simulink model "Practica2"  (R2019a)
settings: Solver=VariableStepAuto  StartTime=0.0  StopTime=10.0  RelTol=1e-3
undefined symbols (not defined in the file or in its folder): k
settings Model: Creator=Andres  LastModifiedBy=Andres

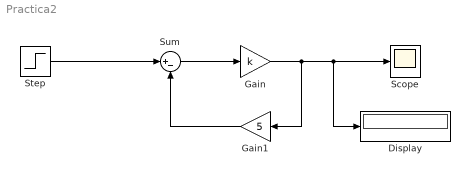
== system Practica2 ==
  Display : Display
  Gain : Gain  Gain=k
  Gain1 : Gain  Gain=5
  Scope : Scope
  Step : Step  SampleTime=0
  Sum : Sum  Inputs=|+-
  wires:
  Sum/1 -> Gain/1
  Step/1 -> Sum/1
  Gain1/1 -> Sum/2
  Gain/1 -> Gain1/1, Display/1, Scope/1
